simulink model "matlabFunction"  (R2016b)
settings: Solver=VariableStepAuto  StartTime=0.0  StopTime=inf  RelTol=1e-3
settings Model: Creator=Hanna Nabil  LastModifiedBy=Hanna Nabil

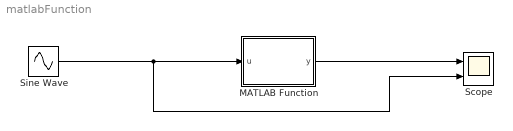
== system matlabFunction ==
  MATLAB Function : MATLAB Function  TreatAsAtomicUnit=on
  Scope : Scope  NumInputPorts=2
  Sine Wave : Sin  SampleTime=0
  wires:
  MATLAB Function/1(y) -> Scope/1
  Sine Wave/1 -> Scope/2, MATLAB Function/1(u)

== matlab function matlabFunction/MATLAB Function ==
  data: u input; y output
function y = fcn(u)

y = u*3+5;
